simulink model "sg_PID_float"  (Simulink 7.8)
settings: Solver=FixedStepDiscrete  SolverMode=SingleTasking  StartTime=0.0  StopTime=1024*II  RelTol=1e-3
PreLoadFcn:
  | sg_PID_float_PreLoadFcn
StopFcn:
  | sg_PID_float_StopFcn
values from neighbouring files (symbols this model uses):
  C = -0.7931    [sg_ClosedLoop_PID_float_PreLoadFcn.m]    (also in sg_PID_float_PreLoadFcn.m)
  Gd = 6.0324    [sg_ClosedLoop_PID_float_PreLoadFcn.m]    (also in sg_PID_float_PreLoadFcn.m)
  Gi = 0.5112    [sg_ClosedLoop_PID_float_PreLoadFcn.m]    (also in sg_PID_float_PreLoadFcn.m)
  Gp = 35.3675    [sg_ClosedLoop_PID_float_PreLoadFcn.m]    (also in sg_PID_float_PreLoadFcn.m)
  II = 37+1    (= 38)    [sg_ClosedLoop_PID_float_PreLoadFcn.m]    (also in sg_PID_float_PreLoadFcn.m)
  max_clip = MAX_VAL-1    (= 255)    [sg_ClosedLoop_PID_float_PreLoadFcn.m]    (also in sg_PID_float_PreLoadFcn.m = 63)
  min_clip = -MAX_VAL    (= -256)    [sg_ClosedLoop_PID_float_PreLoadFcn.m]    (also in sg_PID_float_PreLoadFcn.m = -64)
libraries: xbsIndex_r4 x97, dspsrcs4 x1
settings Model: Creator=danieleb  LastModifiedBy=danieleb

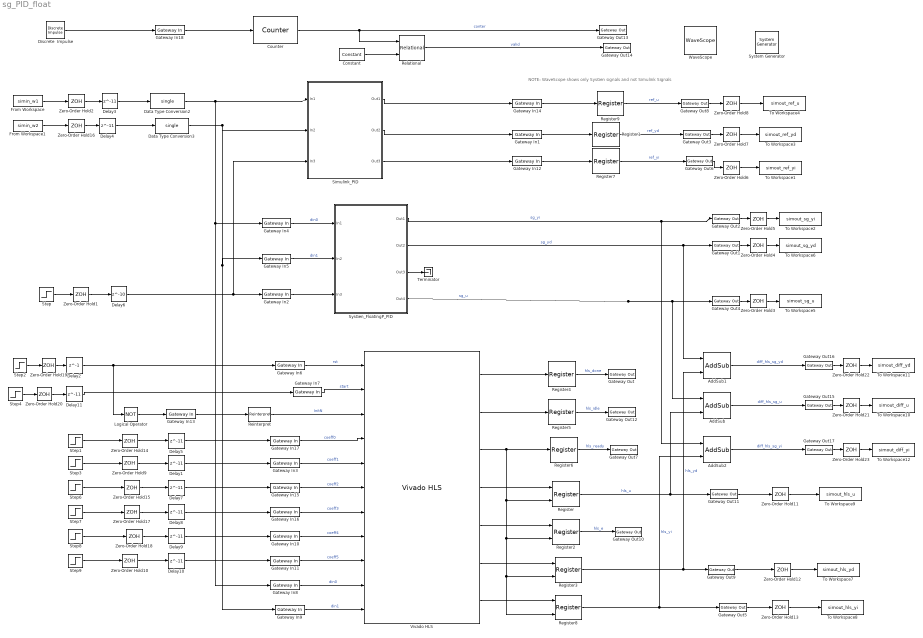
== system sg_PID_float ==
  note: NOTE: WaveScope shows only SysGen signals and not Simulink Signals
  " System Generator" : xbsIndex_r4/ System Generator  Tag=genX  xilinxfamily=zynq  part=xc7z020  speed=-1  package=clg400  synthesis_tool=XST  clock_wrapper=Clock Enables  directory=./netlist_top_PID  proj_type=Project Navigator  Synth_file=XST Defaults  Impl_file=ISE Defaults  testbench=off  simulink_period=1  sysclk_period=10  dcm_input_clock_period=10  incr_netlist=off  trim_vbits=Everywhere in SubSystem  dbl_ovrd=According to Block Masks  core_generation=According to Block Masks  run_coregen=off  deprecated_control=off  eval_field=0  block_type=sysgen
  AddSub : xbsIndex_r4/AddSub  mode=Subtraction  use_carryin=off  use_carryout=off  en=off  latency=0  precision=Full  arith_type=Unsigned  n_bits=16  bin_pt=14  quantization=Truncate  overflow=Wrap  dbl_ovrd=off  use_behavioral_HDL=off  hw_selection=Fabric  pipelined=off  block_type=addsub
  AddSub1 : xbsIndex_r4/AddSub  mode=Subtraction  use_carryin=off  use_carryout=off  en=off  latency=0  precision=Full  arith_type=Unsigned  n_bits=16  bin_pt=14  quantization=Truncate  overflow=Wrap  dbl_ovrd=off  use_behavioral_HDL=off  hw_selection=Fabric  pipelined=off  block_type=addsub
  AddSub2 : xbsIndex_r4/AddSub  mode=Subtraction  use_carryin=off  use_carryout=off  en=off  latency=0  precision=Full  arith_type=Unsigned  n_bits=16  bin_pt=14  quantization=Truncate  overflow=Wrap  dbl_ovrd=off  use_behavioral_HDL=off  hw_selection=Fabric  pipelined=off  block_type=addsub
  Constant : xbsIndex_r4/Constant  const=II-1  gui_display_data_type=Fixed-point  arith_type=Unsigned  n_bits=10  bin_pt=0  preci_type=Single  exp_width=8  frac_width=24  explicit_period=on  period=1  equ=P=C  opselect=C  inp2=PCIN>>17  opr=+  inp1=P  carry=CIN  dbl_ovrd=off  block_type=constant
  Counter : xbsIndex_r4/Counter  cnt_type=Count Limited  cnt_to=II-1  operation=Up  start_count=0  cnt_by_val=1  arith_type=Unsigned  n_bits=10  bin_pt=0  load_pin=off  rst=on  en=off  explicit_period=on  period=1  dbl_ovrd=off  use_behavioral_HDL=off  implementation=Fabric  block_type=counter
  Data Type Conversion2 : DataTypeConversion  OutDataTypeStr=single
  Data Type Conversion3 : DataTypeConversion  OutDataTypeStr=single
  Delay{1,3..5,7..11} (9 alike) : Delay  DelayLength=11
  Delay2 : Delay  DelayLength=1
  Delay6 : Delay  DelayLength=10
  Discrete  Impulse : dspsrcs4/Discrete  Impulse  Delay=0  SampleTime=1  FrameSample=1  dataType=double  isSigned=on  wordLen=16  udDataType=sfix(16)  fracBitsMode=Best precision  numFracBits=15  OutDataTypeStr=double  LastOutDataTypeStr=double
  From Workspace : FromWorkspace  VariableName=simin_w1  SampleTime=II  Interpolate=off  OutputAfterFinalValue=Holding final value
  From Workspace1 : FromWorkspace  VariableName=simin_w2  SampleTime=II  Interpolate=off  OutputAfterFinalValue=Holding final value
  Gateway In{1,3..5,8..12,14..17} (13 alike) : xbsIndex_r4/Gateway In  gui_display_data_type=Floating-point  arith_type=Floating-point  n_bits=25  bin_pt=25-10  preci_type=Single  exp_width=8  frac_width=24  quantization="Round  (unbiased: +/- Inf)"  overflow=Saturate  period=II  dbl_ovrd=off  timing_constraint=None  locs_specified=off  LOCs={}  UseAsADC=off  ADCChannel='1'  inherit_from_input=off  hdl_port=on  block_type=gatewayin
  Gateway In{2,6..7,13} (4 alike) : xbsIndex_r4/Gateway In  gui_display_data_type=Boolean  arith_type=Boolean  n_bits=25  bin_pt=25-10  preci_type=Single  exp_width=8  frac_width=24  quantization="Round  (unbiased: +/- Inf)"  overflow=Saturate  period=II  dbl_ovrd=off  timing_constraint=None  locs_specified=off  LOCs={}  UseAsADC=off  ADCChannel='1'  inherit_from_input=off  hdl_port=on  block_type=gatewayin
  Gateway In18 : xbsIndex_r4/Gateway In  gui_display_data_type=Boolean  arith_type=Boolean  n_bits=25  bin_pt=25-10  preci_type=Single  exp_width=8  frac_width=24  quantization="Round  (unbiased: +/- Inf)"  overflow=Saturate  period=1  dbl_ovrd=off  timing_constraint=None  locs_specified=off  LOCs={}  UseAsADC=off  ADCChannel='1'  inherit_from_input=off  hdl_port=on  block_type=gatewayin
  Gateway Out{,1..6,8..10,12..17} (16 alike) : xbsIndex_r4/Gateway Out  inherit_from_input=off  hdl_port=off  timing_constraint=None  locs_specified=off  LOCs={}  UseAsDAC=off  DACChannel='1'  block_type=gatewayout
  Gateway Out11 : xbsIndex_r4/Gateway Out  inherit_from_input=off  hdl_port=on  timing_constraint=None  locs_specified=off  LOCs={}  UseAsDAC=off  DACChannel='1'  block_type=gatewayout
  Gateway Out7 : xbsIndex_r4/Gateway Out  inherit_from_input=off  hdl_port=on  timing_constraint=None  locs_specified=off  LOCs={}  UseAsDAC=off  DACChannel='1'  block_type=gatewayout
  Logical Operator : Logic  Operator=NOT  AllPortsSameDT=off  OutDataTypeStr=boolean
  Register{,2..3,8} (4 alike) : xbsIndex_r4/Register  init=0  rst=off  en=on  dbl_ovrd=off  block_type=register
  Register{1,4..7,9} (6 alike) : xbsIndex_r4/Register  init=0  rst=off  en=off  dbl_ovrd=off  block_type=register
  Reinterpret : xbsIndex_r4/Reinterpret  force_arith_type=on  arith_type=Unsigned  force_bin_pt=on  bin_pt=0  block_type=reinterpret
  Relational : xbsIndex_r4/Relational  mode=a=b  en=off  latency=0  dbl_ovrd=off  block_type=relational
  Simulink_PID : Subsystem
  Step : Step  Before=1  After=0  SampleTime=II
  Step1 : Step  After=Gi  SampleTime=II
  Step2 : Step  Before=1  After=0  SampleTime=II
  Step3 : Step  After=Gd  SampleTime=II
  Step4 : Step  SampleTime=II
  Step6 : Step  After=C  SampleTime=II
  Step7 : Step  After=Gp  SampleTime=II
  Step8 : Step  After=max_clip  SampleTime=II
  Step9 : Step  After=min_clip  SampleTime=II
  SysGen_FloatingP_PID : Subsystem
      mask Display:
      | fprintf('','COMMENT: begin icon graphics');
      | patch([0 60 60 0 0 ],[0 0 56 56 0 ],[0.77 0.82 0.91 ]);
      | plot([0 60 60 0 0 ],[0 0 56 56 0 ]);
      | patch([12.2 23.76 31.76 39.76 47.76 31.76 20.2 12.2 ],[36.88 36.88 44.88 36.88 44.88 44.88 44.88 36.88 ],[1 1 1 ]);
      | patch([20.2 31.76 23.76 12.2 20.2 ],[28.88 28.88 36.88 36.88 28.88 ],[0.931 0.946 0.973 ]);
      | patch([12.2 23.76 31.76 20.2 12.2 ],[20.88 20.88 28.88 28.88 20.88 ],[1 1 1 ]);
      | patch([20.2 47.76 39.76 31.76 23.76 12.2 20.2 ],[12.88 12.88 20.88 12.88 20.88 20.88 12.88 ],[0.931 0.946 0.973 ]);
      | fprintf('','COMMENT: end icon graphics');
      | fprintf('','COMMENT: begin icon text');
      | color('black');port_label('input',1,' in1');
      | color('black');port_label('input',2,' in2');
      | color('black');port_label('input',3,' rst');
      | color('black');port_label('output',1,'out_i ');
      | color('black');port_label('output',2,'out_d ');
      | color('black');port_label('output',3,'out_p ');
      | color('black');port_label('output',4,'out_u ');
      | fprintf('','COMMENT: end icon text');
  Terminator : Terminator
  To Workspace1 : ToWorkspace  VariableName=simout_ref_yi  SampleTime=-1  SaveFormat=Array
  To Workspace10 : ToWorkspace  VariableName=simout_diff_u  SampleTime=-1  SaveFormat=Array
  To Workspace11 : ToWorkspace  VariableName=simout_diff_yd  SampleTime=-1  SaveFormat=Array
  To Workspace12 : ToWorkspace  VariableName=simout_diff_yi  SampleTime=-1  SaveFormat=Array
  To Workspace2 : ToWorkspace  VariableName=simout_sg_yi  SampleTime=-1  SaveFormat=Array
  To Workspace3 : ToWorkspace  VariableName=simout_ref_yd  SampleTime=-1  SaveFormat=Array
  To Workspace4 : ToWorkspace  VariableName=simout_ref_u  SampleTime=-1  SaveFormat=Array
  To Workspace5 : ToWorkspace  VariableName=simout_sg_u  SampleTime=-1  SaveFormat=Array
  To Workspace6 : ToWorkspace  VariableName=simout_sg_yd  SampleTime=-1  SaveFormat=Array
  To Workspace7 : ToWorkspace  VariableName=simout_hls_yd  SampleTime=-1  SaveFormat=Array
  To Workspace8 : ToWorkspace  VariableName=simout_hls_yi  SampleTime=-1  SaveFormat=Array
  To Workspace9 : ToWorkspace  VariableName=simout_hls_u  SampleTime=-1  SaveFormat=Array
  Vivado HLS : xbsIndex_r4/Vivado HLS  anytable='C:/BagniD/work/xapp_pid/hls/floatp/hls_floatp_pid_prj/solution3_test/'  display_datatype=off  rate_propagation_method=Simulink system period  model_file_path=''  latency=1  block_type=hls
      settings: infoedit=This block allows including C,C++ and SystemC source files in System Generator for DSP designs.
  WaveScope : xbsIndex_r4/WaveScope  block_type=wavescope
  Zero-Order Hold{1..8,11..13,16,19..23} (17 alike) : ZeroOrderHold  SampleTime=II
  Zero-Order Hold{9..10,14..15,17..18} (6 alike) : ZeroOrderHold  SampleTime=-1
  wires:
  Gateway In4/1 -> SysGen_FloatingP_PID/1(In1)  "din0"
  Gateway In5/1 -> SysGen_FloatingP_PID/2(In2)  "din1"
  Register7/1 -> Gateway Out6/1  "ref_yi"
  Gateway In12/1 -> Register7/1
  Gateway Out6/1 -> Zero-Order Hold6/1
  Gateway Out8/1 -> Zero-Order Hold8/1
  Gateway In14/1 -> Register9/1
  Simulink_PID/1(Out1) -> Gateway In14/1
  Register9/1 -> Gateway Out8/1  "ref_u"
  Gateway Out1/1 -> Zero-Order Hold4/1
  Gateway Out2/1 -> Zero-Order Hold5/1
  Gateway Out4/1 -> Zero-Order Hold3/1
  SysGen_FloatingP_PID/4(Out4) -> Gateway Out4/1, AddSub/1  "sg_u"
  Data Type Conversion2/1 -> Gateway In4/1, Gateway In8/1, Simulink_PID/1(In1)
  Data Type Conversion3/1 -> Gateway In5/1, Gateway In9/1, Simulink_PID/2(In2)
  SysGen_FloatingP_PID/1(Out1) -> Gateway Out2/1, AddSub2/1  "sg_yi"
  SysGen_FloatingP_PID/2(Out2) -> Gateway Out1/1, AddSub1/1  "sg_yd"
  SysGen_FloatingP_PID/3(Out3) -> Terminator/1
  Register1/1 -> Gateway Out3/1  "ref_yd"
  Gateway Out3/1 -> Zero-Order Hold7/1
  Gateway In1/1 -> Register1/1
  Gateway In2/1 -> SysGen_FloatingP_PID/3(In3)
  Step/1 -> Zero-Order Hold1/1
  Zero-Order Hold1/1 -> Delay6/1
  Delay6/1 -> Gateway In2/1, Simulink_PID/3(In3)
  Delay3/1 -> Data Type Conversion2/1
  Zero-Order Hold16/1 -> Delay4/1
  Delay4/1 -> Data Type Conversion3/1
  Zero-Order Hold2/1 -> Delay3/1
  From Workspace/1 -> Zero-Order Hold2/1
  From Workspace1/1 -> Zero-Order Hold16/1
  Zero-Order Hold3/1 -> To Workspace5/1
  Zero-Order Hold4/1 -> To Workspace6/1
  Zero-Order Hold5/1 -> To Workspace2/1
  Zero-Order Hold6/1 -> To Workspace1/1
  Zero-Order Hold7/1 -> To Workspace3/1
  Zero-Order Hold8/1 -> To Workspace4/1
  Gateway In6/1 -> Vivado HLS/1  "rst"
  Delay2/1 -> Gateway In6/1, Logical Operator/1
  Delay11/1 -> Gateway In7/1
  Delay5/1 -> Gateway In17/1
  Gateway In17/1 -> Vivado HLS/4  "coeff0"
  Gateway In7/1 -> Vivado HLS/2  "start"
  Reinterpret/1 -> Vivado HLS/3  "InitN"
  Zero-Order Hold14/1 -> Delay5/1
  Step1/1 -> Zero-Order Hold14/1
  Delay1/1 -> Gateway In3/1
  Gateway In3/1 -> Vivado HLS/5  "coeff1"
  Zero-Order Hold9/1 -> Delay1/1
  Step3/1 -> Zero-Order Hold9/1
  Gateway In8/1 -> Vivado HLS/10  "din0"
  Gateway In9/1 -> Vivado HLS/11  "din1"
  Gateway In13/1 -> Reinterpret/1
  Logical Operator/1 -> Gateway In13/1
  Gateway In15/1 -> Vivado HLS/6  "coeff2"
  Gateway In16/1 -> Vivado HLS/7  "coeff3"
  Gateway In10/1 -> Vivado HLS/8  "coeff4"
  Gateway In11/1 -> Vivado HLS/9  "coeff5"
  Delay7/1 -> Gateway In15/1
  Delay8/1 -> Gateway In16/1
  Delay9/1 -> Gateway In10/1
  Delay10/1 -> Gateway In11/1
  Zero-Order Hold15/1 -> Delay7/1
  Zero-Order Hold17/1 -> Delay8/1
  Step6/1 -> Zero-Order Hold15/1
  Step7/1 -> Zero-Order Hold17/1
  Zero-Order Hold18/1 -> Delay9/1
  Step8/1 -> Zero-Order Hold18/1
  Zero-Order Hold10/1 -> Delay10/1
  Step9/1 -> Zero-Order Hold10/1
  Register/1 -> Gateway Out11/1, AddSub/2  "hls_u"
  Register2/1 -> Gateway Out10/1  "hls_e"
  Register3/1 -> Gateway Out9/1, AddSub1/2  "hls_yd"
  Register4/1 -> Gateway Out/1  "hls_done"
  Register5/1 -> Gateway Out12/1  "hls_idle"
  Register6/1 -> Gateway Out7/1  "hls_ready"
  Register8/1 -> Gateway Out5/1, AddSub2/2  "hls_yi"
  Gateway Out9/1 -> Zero-Order Hold12/1
  Gateway Out5/1 -> Zero-Order Hold13/1
  Gateway Out11/1 -> Zero-Order Hold11/1
  Vivado HLS/1 -> Register4/1
  Vivado HLS/2 -> Register5/1
  Vivado HLS/3 -> Register6/1, Register/2, Register2/2, Register3/2, Register8/2
  Vivado HLS/4 -> Register/1
  Vivado HLS/5 -> Register2/1
  Vivado HLS/6 -> Register3/1
  Vivado HLS/7 -> Register8/1
  Zero-Order Hold11/1 -> To Workspace9/1
  Zero-Order Hold12/1 -> To Workspace7/1
  Zero-Order Hold13/1 -> To Workspace8/1
  Step2/1 -> Zero-Order Hold19/1
  Zero-Order Hold19/1 -> Delay2/1
  Step4/1 -> Zero-Order Hold20/1
  Zero-Order Hold20/1 -> Delay11/1
  Gateway In18/1 -> Counter/1
  Discrete  Impulse/1 -> Gateway In18/1
  Counter/1 -> Gateway Out13/1, Relational/1  "conter"
  Constant/1 -> Relational/2
  Relational/1 -> Gateway Out14/1  "valid"
  Gateway Out15/1 -> Zero-Order Hold21/1
  AddSub/1 -> Gateway Out15/1  "diff_hls_sg_u"
  Zero-Order Hold21/1 -> To Workspace10/1
  Gateway Out16/1 -> Zero-Order Hold22/1
  AddSub1/1 -> Gateway Out16/1  "diff_hls_sg_yd"
  Zero-Order Hold22/1 -> To Workspace11/1
  Gateway Out17/1 -> Zero-Order Hold23/1
  AddSub2/1 -> Gateway Out17/1  "diff_hls_sg_yi"
  Zero-Order Hold23/1 -> To Workspace12/1
  Simulink_PID/2(Out2) -> Gateway In1/1
  Simulink_PID/3(Out3) -> Gateway In12/1

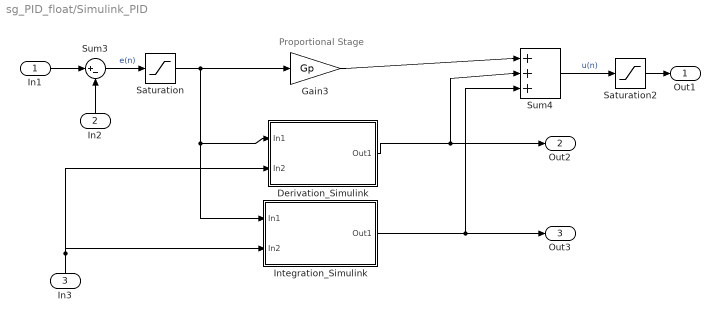
== system sg_PID_float/Simulink_PID ==
  note: Proportional Stage
  In1 : Inport
  In2 : Inport  Port=2
  In3 : Inport  Port=3
  Derivation_Simulink : Subsystem
  Gain3 : Gain  Gain=Gp
  Integration_Simulink : Subsystem
  Saturation : Saturate  UpperLimit=max_clip  LowerLimit=min_clip
  Saturation2 : Saturate  UpperLimit=max_clip  LowerLimit=min_clip
  Sum3 : Sum  Inputs=|+-
  Sum4 : Sum  Inputs=|+++
  Out1 : Outport
  Out2 : Outport  Port=2
  Out3 : Outport  Port=3
  wires:
  Gain3/1 -> Sum4/1
  Sum3/1 -> Saturation/1  "e(n)"
  Sum4/1 -> Saturation2/1  "u(n)"
  Saturation/1 -> Gain3/1, Derivation_Simulink/1(In1), Integration_Simulink/1(In1)
  Derivation_Simulink/1(Out1) -> Sum4/2, Out2/1
  Integration_Simulink/1(Out1) -> Sum4/3, Out3/1
  In1/1 -> Sum3/1
  In2/1 -> Sum3/2
  In3/1 -> Integration_Simulink/2(In2), Derivation_Simulink/2(In2)
  Saturation2/1 -> Out1/1

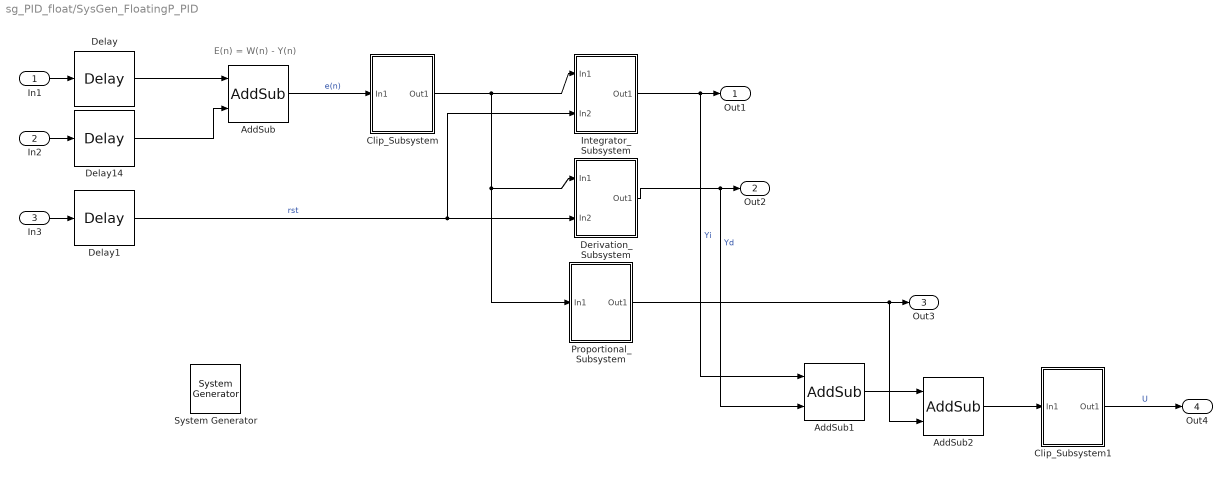
== system sg_PID_float/SysGen_FloatingP_PID ==
  note: E(n) = W(n) - Y(n)
  In1 : Inport
  In2 : Inport  Port=2
  In3 : Inport  Port=3
  " System Generator" : xbsIndex_r4/ System Generator  Tag=genX  xilinxfamily=virtex6  part=xc6vlx240t  speed=-2  package=ff1156  synthesis_tool=XST  clock_wrapper=Clock Enables  directory=./timing_v6lx240t  proj_type=Project Navigator  Synth_file=XST Defaults  Impl_file=ISE Defaults  testbench=off  simulink_period=1  sysclk_period=1.000000e+001  dcm_input_clock_period=10  incr_netlist=off  trim_vbits=Everywhere in SubSystem  dbl_ovrd=According to Block Masks  core_generation=According to Block Masks  run_coregen=off  deprecated_control=off  eval_field=0  block_type=sysgen
  AddSub : xbsIndex_r4/AddSub  mode=Subtraction  use_carryin=off  use_carryout=off  en=off  latency=0  precision=Full  arith_type=Unsigned  n_bits=16  bin_pt=14  quantization=Truncate  overflow=Wrap  dbl_ovrd=off  use_behavioral_HDL=off  hw_selection=DSP48  pipelined=off  block_type=addsub
  AddSub1 : xbsIndex_r4/AddSub  mode=Addition  use_carryin=off  use_carryout=off  en=off  latency=0  precision=Full  arith_type=Unsigned  n_bits=16  bin_pt=14  quantization=Truncate  overflow=Wrap  dbl_ovrd=off  use_behavioral_HDL=off  hw_selection=DSP48  pipelined=off  block_type=addsub
  AddSub2 : xbsIndex_r4/AddSub  mode=Addition  use_carryin=off  use_carryout=off  en=off  latency=0  precision=Full  arith_type=Unsigned  n_bits=16  bin_pt=14  quantization=Truncate  overflow=Wrap  dbl_ovrd=off  use_behavioral_HDL=off  hw_selection=DSP48  pipelined=off  block_type=addsub
  Clip_Subsystem : Subsystem
      mask Display:
      | fprintf('','COMMENT: begin icon graphics');
      | patch([0 60 60 0 0 ],[0 0 58 58 0 ],[0.77 0.82 0.91 ]);
      | plot([0 60 60 0 0 ],[0 0 58 58 0 ]);
      | patch([12.2 23.76 31.76 39.76 47.76 31.76 20.2 12.2 ],[37.88 37.88 45.88 37.88 45.88 45.88 45.88 37.88 ],[1 1 1 ]);
      | patch([20.2 31.76 23.76 12.2 20.2 ],[29.88 29.88 37.88 37.88 29.88 ],[0.931 0.946 0.973 ]);
      | patch([12.2 23.76 31.76 20.2 12.2 ],[21.88 21.88 29.88 29.88 21.88 ],[1 1 1 ]);
      | patch([20.2 47.76 39.76 31.76 23.76 12.2 20.2 ],[13.88 13.88 21.88 13.88 21.88 21.88 13.88 ],[0.931 0.946 0.973 ]);
      | fprintf('','COMMENT: end icon graphics');
      | fprintf('','COMMENT: begin icon text');
      | color('black');port_label('input',1,' Din');
      | color('black');port_label('output',1,'Dout ');
      | fprintf('','COMMENT: end icon text');
  Clip_Subsystem1 : Subsystem
      mask Display:
      | fprintf('','COMMENT: begin icon graphics');
      | patch([0 60 60 0 0 ],[0 0 58 58 0 ],[0.77 0.82 0.91 ]);
      | plot([0 60 60 0 0 ],[0 0 58 58 0 ]);
      | patch([12.2 23.76 31.76 39.76 47.76 31.76 20.2 12.2 ],[37.88 37.88 45.88 37.88 45.88 45.88 45.88 37.88 ],[1 1 1 ]);
      | patch([20.2 31.76 23.76 12.2 20.2 ],[29.88 29.88 37.88 37.88 29.88 ],[0.931 0.946 0.973 ]);
      | patch([12.2 23.76 31.76 20.2 12.2 ],[21.88 21.88 29.88 29.88 21.88 ],[1 1 1 ]);
      | patch([20.2 47.76 39.76 31.76 23.76 12.2 20.2 ],[13.88 13.88 21.88 13.88 21.88 21.88 13.88 ],[0.931 0.946 0.973 ]);
      | fprintf('','COMMENT: end icon graphics');
      | fprintf('','COMMENT: begin icon text');
      | color('black');port_label('input',1,' Din');
      | color('black');port_label('output',1,'Dout ');
      | fprintf('','COMMENT: end icon text');
  Delay : xbsIndex_r4/Delay  rst=off  infoeditControl=Selection of Reset will increase slice count due to use of real FFs and instead of SRLs  en=off  latency=1  dbl_ovrd=off  reg_retiming=off  block_type=delay
  Delay1 : xbsIndex_r4/Delay  rst=off  infoeditControl=Selection of Reset will increase slice count due to use of real FFs and instead of SRLs  en=off  latency=1  dbl_ovrd=off  reg_retiming=off  block_type=delay
  Delay14 : xbsIndex_r4/Delay  rst=off  infoeditControl=Selection of Reset will increase slice count due to use of real FFs and instead of SRLs  en=off  latency=1  dbl_ovrd=off  reg_retiming=off  block_type=delay
  Derivation_Subsystem : Subsystem
      mask Display:
      | fprintf('','COMMENT: begin icon graphics');
      | patch([0 60 60 0 0 ],[0 0 58 58 0 ],[0.77 0.82 0.91 ]);
      | plot([0 60 60 0 0 ],[0 0 58 58 0 ]);
      | patch([12.2 23.76 31.76 39.76 47.76 31.76 20.2 12.2 ],[37.88 37.88 45.88 37.88 45.88 45.88 45.88 37.88 ],[1 1 1 ]);
      | patch([20.2 31.76 23.76 12.2 20.2 ],[29.88 29.88 37.88 37.88 29.88 ],[0.931 0.946 0.973 ]);
      | patch([12.2 23.76 31.76 20.2 12.2 ],[21.88 21.88 29.88 29.88 21.88 ],[1 1 1 ]);
      | patch([20.2 47.76 39.76 31.76 23.76 12.2 20.2 ],[13.88 13.88 21.88 13.88 21.88 21.88 13.88 ],[0.931 0.946 0.973 ]);
      | fprintf('','COMMENT: end icon graphics');
      | fprintf('','COMMENT: begin icon text');
      | color('black');port_label('input',1,' X1');
      | color('black');port_label('output',1,'Yd ');
      | fprintf('','COMMENT: end icon text');
  Integrator_Subsystem : Subsystem
      mask Display:
      | fprintf('','COMMENT: begin icon graphics');
      | patch([0 60 60 0 0 ],[0 0 58 58 0 ],[0.77 0.82 0.91 ]);
      | plot([0 60 60 0 0 ],[0 0 58 58 0 ]);
      | patch([12.2 23.76 31.76 39.76 47.76 31.76 20.2 12.2 ],[37.88 37.88 45.88 37.88 45.88 45.88 45.88 37.88 ],[1 1 1 ]);
      | patch([20.2 31.76 23.76 12.2 20.2 ],[29.88 29.88 37.88 37.88 29.88 ],[0.931 0.946 0.973 ]);
      | patch([12.2 23.76 31.76 20.2 12.2 ],[21.88 21.88 29.88 29.88 21.88 ],[1 1 1 ]);
      | patch([20.2 47.76 39.76 31.76 23.76 12.2 20.2 ],[13.88 13.88 21.88 13.88 21.88 21.88 13.88 ],[0.931 0.946 0.973 ]);
      | fprintf('','COMMENT: end icon graphics');
      | fprintf('','COMMENT: begin icon text');
      | color('black');port_label('input',1,' X2');
      | color('black');port_label('output',1,'Yi ');
      | fprintf('','COMMENT: end icon text');
  Proportional_Subsystem : Subsystem
      mask Display:
      | fprintf('','COMMENT: begin icon graphics');
      | patch([0 60 60 0 0 ],[0 0 58 58 0 ],[0.77 0.82 0.91 ]);
      | plot([0 60 60 0 0 ],[0 0 58 58 0 ]);
      | patch([12.2 23.76 31.76 39.76 47.76 31.76 20.2 12.2 ],[37.88 37.88 45.88 37.88 45.88 45.88 45.88 37.88 ],[1 1 1 ]);
      | patch([20.2 31.76 23.76 12.2 20.2 ],[29.88 29.88 37.88 37.88 29.88 ],[0.931 0.946 0.973 ]);
      | patch([12.2 23.76 31.76 20.2 12.2 ],[21.88 21.88 29.88 29.88 21.88 ],[1 1 1 ]);
      | patch([20.2 47.76 39.76 31.76 23.76 12.2 20.2 ],[13.88 13.88 21.88 13.88 21.88 21.88 13.88 ],[0.931 0.946 0.973 ]);
      | fprintf('','COMMENT: end icon graphics');
      | fprintf('','COMMENT: begin icon text');
      | color('black');port_label('input',1,' X');
      | color('black');port_label('output',1,'Y ');
      | fprintf('','COMMENT: end icon text');
  Out1 : Outport
  Out2 : Outport  Port=2
  Out3 : Outport  Port=3
  Out4 : Outport  Port=4
  wires:
  Delay/1 -> AddSub/1
  Delay14/1 -> AddSub/2
  AddSub/1 -> Clip_Subsystem/1(In1)  "e(n)"
  Clip_Subsystem/1(Out1) -> Integrator_Subsystem/1(In1), Derivation_Subsystem/1(In1), Proportional_Subsystem/1(In1)
  Derivation_Subsystem/1(Out1) -> AddSub1/2, Out2/1  "Yd"
  Integrator_Subsystem/1(Out1) -> AddSub1/1, Out1/1  "Yi"
  Proportional_Subsystem/1(Out1) -> AddSub2/2, Out3/1
  AddSub1/1 -> AddSub2/1
  AddSub2/1 -> Clip_Subsystem1/1(In1)
  In1/1 -> Delay/1
  In2/1 -> Delay14/1
  Clip_Subsystem1/1(Out1) -> Out4/1  "U"
  In3/1 -> Delay1/1
  Delay1/1 -> Integrator_Subsystem/2(In2), Derivation_Subsystem/2(In2)  "rst"

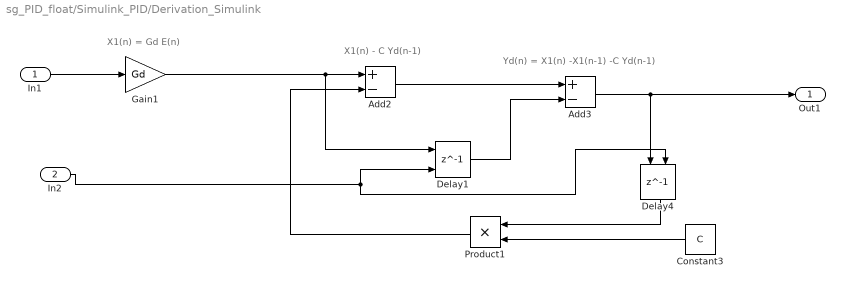
== system sg_PID_float/Simulink_PID/Derivation_Simulink ==
  note: X1(n) - C Yd(n-1)
  note: Yd(n) = X1(n) -X1(n-1) -C Yd(n-1)
  note: X1(n) = Gd E(n)
  In1 : Inport
  In2 : Inport  Port=2
  Add2 : Sum  Inputs=+-
  Add3 : Sum  Inputs=+-
  Constant3 : Constant  Value=C  OutDataTypeStr=single  SampleTime=II
  Delay1 : Delay  DelayLength=1  ExternalReset=Level hold
      settings: InputPortMap=u0,r5
  Delay4 : Delay  DelayLength=1  ExternalReset=Level hold
      settings: InputPortMap=u0,r5
  Gain1 : Gain  Gain=Gd
  Product1 : Product  RndMeth=Zero
  Out1 : Outport
  wires:
  In1/1 -> Gain1/1
  Delay1/1 -> Add3/2
  Add2/1 -> Add3/1
  Add3/1 -> Delay4/1, Out1/1
  Constant3/1 -> Product1/2
  Product1/1 -> Add2/2
  Delay4/1 -> Product1/1
  In2/1 -> Delay1/2, Delay4/2
  Gain1/1 -> Add2/1, Delay1/1

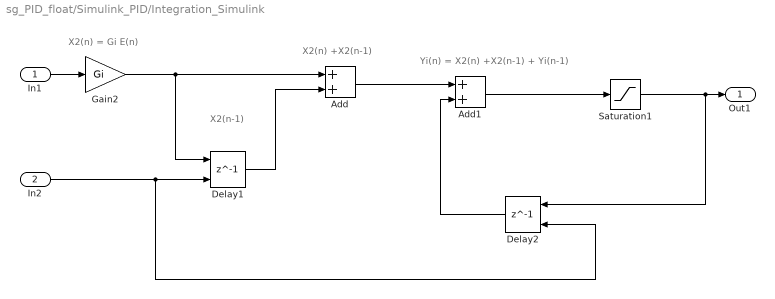
== system sg_PID_float/Simulink_PID/Integration_Simulink ==
  note: X2(n) = Gi E(n)
  note: X2(n) +X2(n-1)
  note: X2(n-1)
  note: Yi(n) = X2(n) +X2(n-1) + Yi(n-1)
  In1 : Inport
  In2 : Inport  Port=2
  Add : Sum
  Add1 : Sum
  Delay1 : Delay  DelayLength=1  ExternalReset=Level hold
      settings: InputPortMap=u0,r5
  Delay2 : Delay  DelayLength=1  ExternalReset=Level hold
      settings: InputPortMap=u0,r5
  Gain2 : Gain  Gain=Gi
  Saturation1 : Saturate  UpperLimit=max_clip  LowerLimit=min_clip
  Out1 : Outport
  wires:
  Add/1 -> Add1/1
  Add1/1 -> Saturation1/1
  Gain2/1 -> Add/1, Delay1/1
  Delay1/1 -> Add/2
  Saturation1/1 -> Out1/1, Delay2/1
  In1/1 -> Gain2/1
  Delay2/1 -> Add1/2
  In2/1 -> Delay1/2, Delay2/2

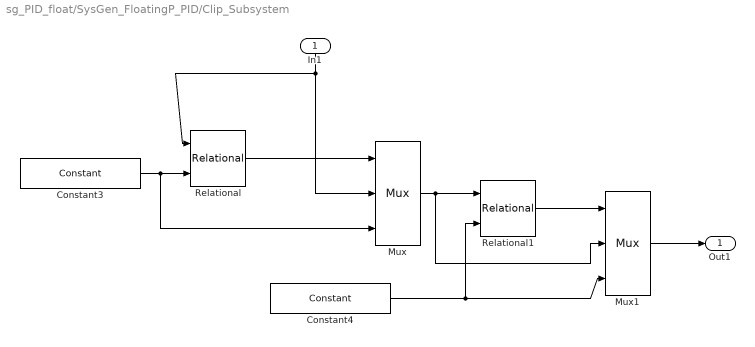
== system sg_PID_float/SysGen_FloatingP_PID/Clip_Subsystem ==
  In1 : Inport
  Constant3 : xbsIndex_r4/Constant  const=max_clip  gui_display_data_type=Floating-point  arith_type=Floating-point  n_bits=16  bin_pt=14  preci_type=Single  exp_width=8  frac_width=24  explicit_period=on  period=II  equ=P=C  opselect=C  inp2=PCIN>>17  opr=+  inp1=P  carry=CIN  dbl_ovrd=off  block_type=constant
  Constant4 : xbsIndex_r4/Constant  const=min_clip  gui_display_data_type=Floating-point  arith_type=Floating-point  n_bits=16  bin_pt=14  preci_type=Single  exp_width=8  frac_width=24  explicit_period=on  period=II  equ=P=C  opselect=C  inp2=PCIN>>17  opr=+  inp1=P  carry=CIN  dbl_ovrd=off  block_type=constant
  Mux : xbsIndex_r4/Mux  inputs=2  en=off  latency=0  precision=Full  arith_type=Unsigned  n_bits=16  bin_pt=14  quantization=Truncate  overflow=Wrap  dbl_ovrd=off  block_type=mux
  Mux1 : xbsIndex_r4/Mux  inputs=2  en=off  latency=0  precision=Full  arith_type=Unsigned  n_bits=16  bin_pt=14  quantization=Truncate  overflow=Wrap  dbl_ovrd=off  block_type=mux
  Relational : xbsIndex_r4/Relational  mode=a>=b  en=off  latency=0  dbl_ovrd=off  block_type=relational
  Relational1 : xbsIndex_r4/Relational  mode=a<=b  en=off  latency=0  dbl_ovrd=off  block_type=relational
  Out1 : Outport
  wires:
  Constant3/1 -> Relational/2, Mux/3
  Relational/1 -> Mux/1
  In1/1 -> Relational/1, Mux/2
  Mux/1 -> Relational1/1, Mux1/2
  Constant4/1 -> Mux1/3, Relational1/2
  Relational1/1 -> Mux1/1
  Mux1/1 -> Out1/1

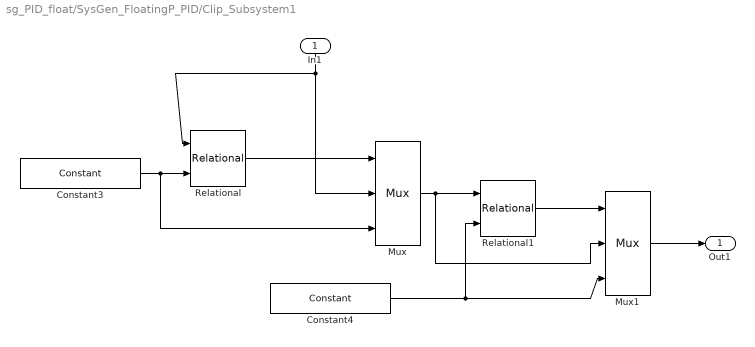
== system sg_PID_float/SysGen_FloatingP_PID/Clip_Subsystem1 ==
  In1 : Inport
  Constant3 : xbsIndex_r4/Constant  const=max_clip  gui_display_data_type=Floating-point  arith_type=Floating-point  n_bits=16  bin_pt=14  preci_type=Single  exp_width=8  frac_width=24  explicit_period=on  period=II  equ=P=C  opselect=C  inp2=PCIN>>17  opr=+  inp1=P  carry=CIN  dbl_ovrd=off  block_type=constant
  Constant4 : xbsIndex_r4/Constant  const=min_clip  gui_display_data_type=Floating-point  arith_type=Floating-point  n_bits=16  bin_pt=14  preci_type=Single  exp_width=8  frac_width=24  explicit_period=on  period=II  equ=P=C  opselect=C  inp2=PCIN>>17  opr=+  inp1=P  carry=CIN  dbl_ovrd=off  block_type=constant
  Mux : xbsIndex_r4/Mux  inputs=2  en=off  latency=0  precision=Full  arith_type=Unsigned  n_bits=16  bin_pt=14  quantization=Truncate  overflow=Wrap  dbl_ovrd=off  block_type=mux
  Mux1 : xbsIndex_r4/Mux  inputs=2  en=off  latency=0  precision=Full  arith_type=Unsigned  n_bits=16  bin_pt=14  quantization=Truncate  overflow=Wrap  dbl_ovrd=off  block_type=mux
  Relational : xbsIndex_r4/Relational  mode=a>=b  en=off  latency=0  dbl_ovrd=off  block_type=relational
  Relational1 : xbsIndex_r4/Relational  mode=a<=b  en=off  latency=0  dbl_ovrd=off  block_type=relational
  Out1 : Outport
  wires:
  Mux1/1 -> Out1/1
  Relational1/1 -> Mux1/1
  Constant4/1 -> Relational1/2, Mux1/3
  Mux/1 -> Mux1/2, Relational1/1
  In1/1 -> Mux/2, Relational/1
  Relational/1 -> Mux/1
  Constant3/1 -> Mux/3, Relational/2

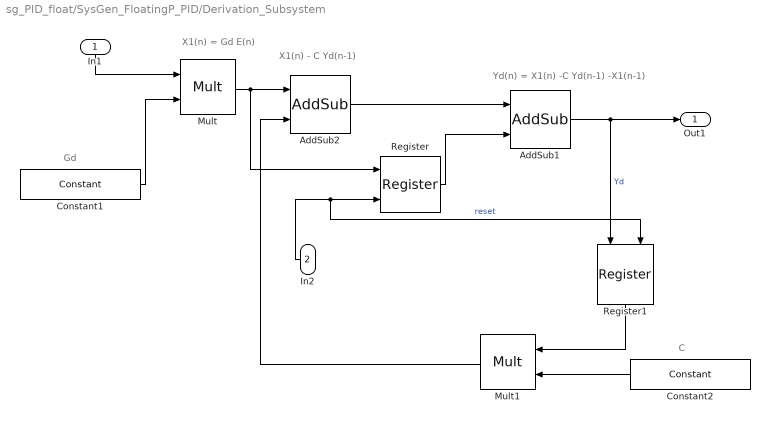
== system sg_PID_float/SysGen_FloatingP_PID/Derivation_Subsystem ==
  note: X1(n) - C Yd(n-1)
  note: Yd(n) = X1(n) -C Yd(n-1) -X1(n-1)
  note: X1(n) = Gd E(n)
  note: Gd
  note: C
  In1 : Inport
  In2 : Inport  Port=2
  AddSub1 : xbsIndex_r4/AddSub  mode=Subtraction  use_carryin=off  use_carryout=off  en=off  latency=0  precision=Full  arith_type=Unsigned  n_bits=16  bin_pt=14  quantization=Truncate  overflow=Wrap  dbl_ovrd=off  use_behavioral_HDL=off  hw_selection=Fabric  pipelined=off  block_type=addsub
  AddSub2 : xbsIndex_r4/AddSub  mode=Subtraction  use_carryin=off  use_carryout=off  en=off  latency=0  precision=Full  arith_type=Unsigned  n_bits=16  bin_pt=14  quantization=Truncate  overflow=Wrap  dbl_ovrd=off  use_behavioral_HDL=off  hw_selection=Fabric  pipelined=off  block_type=addsub
  Constant1 : xbsIndex_r4/Constant  const=Gd  gui_display_data_type=Floating-point  arith_type=Floating-point  n_bits=16  bin_pt=14  preci_type=Single  exp_width=8  frac_width=24  explicit_period=on  period=II  equ=P=C  opselect=C  inp2=PCIN>>17  opr=+  inp1=P  carry=CIN  dbl_ovrd=off  block_type=constant
  Constant2 : xbsIndex_r4/Constant  const=C  gui_display_data_type=Floating-point  arith_type=Floating-point  n_bits=16  bin_pt=14  preci_type=Single  exp_width=8  frac_width=24  explicit_period=on  period=II  equ=P=C  opselect=C  inp2=PCIN>>17  opr=+  inp1=P  carry=CIN  dbl_ovrd=off  block_type=constant
  Mult : xbsIndex_r4/Mult  precision=Full  arith_type="Signed  (2's comp)"  n_bits=16  bin_pt=14  quantization=Truncate  overflow=Wrap  en=off  latency=0  dbl_ovrd=off  use_behavioral_HDL=off  opt=Speed  use_embedded=on  optimum_pipeline=off  pipeline=on  use_rpm=on  placement_style=Triangular  block_type=mult
  Mult1 : xbsIndex_r4/Mult  precision=Full  arith_type="Signed  (2's comp)"  n_bits=16  bin_pt=14  quantization=Truncate  overflow=Wrap  en=off  latency=0  dbl_ovrd=off  use_behavioral_HDL=off  opt=Speed  use_embedded=on  optimum_pipeline=off  pipeline=on  use_rpm=on  placement_style=Triangular  block_type=mult
  Register : xbsIndex_r4/Register  init=0  rst=on  en=off  dbl_ovrd=off  block_type=register
  Register1 : xbsIndex_r4/Register  init=0  rst=on  en=off  dbl_ovrd=off  block_type=register
  Out1 : Outport
  wires:
  In1/1 -> Mult/1
  AddSub2/1 -> AddSub1/1
  Mult/1 -> AddSub2/1, Register/1
  Mult1/1 -> AddSub2/2
  Constant2/1 -> Mult1/2
  AddSub1/1 -> Out1/1, Register1/1  "Yd"
  Register/1 -> AddSub1/2
  Constant1/1 -> Mult/2
  Register1/1 -> Mult1/1
  In2/1 -> Register/2, Register1/2  "reset"

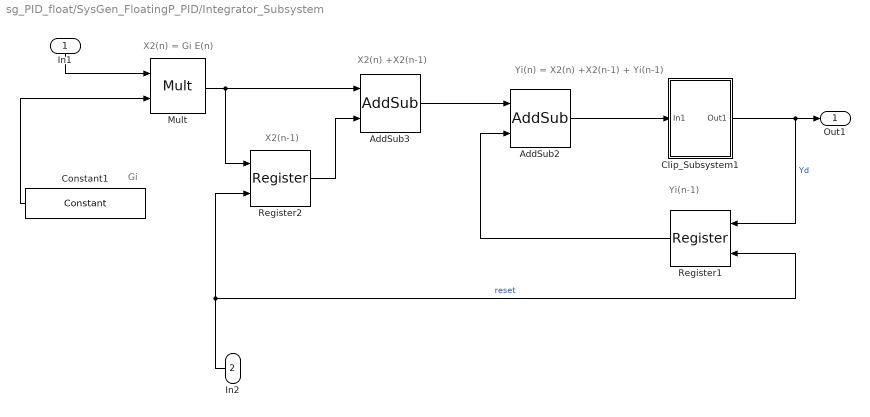
== system sg_PID_float/SysGen_FloatingP_PID/Integrator_Subsystem ==
  note: X2(n) = Gi E(n)
  note: Yi(n) = X2(n) +X2(n-1) + Yi(n-1)
  note: X2(n) +X2(n-1)
  note: X2(n-1)
  note: Yi(n-1)
  note: Gi
  In1 : Inport
  In2 : Inport  Port=2
  AddSub2 : xbsIndex_r4/AddSub  mode=Addition  use_carryin=off  use_carryout=off  en=off  latency=0  precision=Full  arith_type=Unsigned  n_bits=16  bin_pt=14  quantization=Truncate  overflow=Wrap  dbl_ovrd=off  use_behavioral_HDL=off  hw_selection=DSP48  pipelined=off  block_type=addsub
  AddSub3 : xbsIndex_r4/AddSub  mode=Addition  use_carryin=off  use_carryout=off  en=off  latency=0  precision=Full  arith_type=Unsigned  n_bits=16  bin_pt=14  quantization=Truncate  overflow=Wrap  dbl_ovrd=off  use_behavioral_HDL=off  hw_selection=DSP48  pipelined=off  block_type=addsub
  Clip_Subsystem1 : Subsystem
      mask Display:
      | fprintf('','COMMENT: begin icon graphics');
      | patch([0 60 60 0 0 ],[0 0 58 58 0 ],[0.77 0.82 0.91 ]);
      | plot([0 60 60 0 0 ],[0 0 58 58 0 ]);
      | patch([12.2 23.76 31.76 39.76 47.76 31.76 20.2 12.2 ],[37.88 37.88 45.88 37.88 45.88 45.88 45.88 37.88 ],[1 1 1 ]);
      | patch([20.2 31.76 23.76 12.2 20.2 ],[29.88 29.88 37.88 37.88 29.88 ],[0.931 0.946 0.973 ]);
      | patch([12.2 23.76 31.76 20.2 12.2 ],[21.88 21.88 29.88 29.88 21.88 ],[1 1 1 ]);
      | patch([20.2 47.76 39.76 31.76 23.76 12.2 20.2 ],[13.88 13.88 21.88 13.88 21.88 21.88 13.88 ],[0.931 0.946 0.973 ]);
      | fprintf('','COMMENT: end icon graphics');
      | fprintf('','COMMENT: begin icon text');
      | color('black');port_label('input',1,' Din');
      | color('black');port_label('output',1,'Dout ');
      | fprintf('','COMMENT: end icon text');
  Constant1 : xbsIndex_r4/Constant  const=Gi  gui_display_data_type=Floating-point  arith_type=Floating-point  n_bits=16  bin_pt=14  preci_type=Single  exp_width=8  frac_width=24  explicit_period=on  period=II  equ=P=C  opselect=C  inp2=PCIN>>17  opr=+  inp1=P  carry=CIN  dbl_ovrd=off  block_type=constant
  Mult : xbsIndex_r4/Mult  precision=Full  arith_type="Signed  (2's comp)"  n_bits=16  bin_pt=14  quantization=Truncate  overflow=Wrap  en=off  latency=0  dbl_ovrd=off  use_behavioral_HDL=off  opt=Speed  use_embedded=on  optimum_pipeline=off  pipeline=on  use_rpm=on  placement_style=Triangular  block_type=mult
  Register1 : xbsIndex_r4/Register  init=0  rst=on  en=off  dbl_ovrd=off  block_type=register
  Register2 : xbsIndex_r4/Register  init=0  rst=on  en=off  dbl_ovrd=off  block_type=register
  Out1 : Outport
  wires:
  Constant1/1 -> Mult/2
  Clip_Subsystem1/1(Out1) -> Out1/1, Register1/1  "Yd"
  In1/1 -> Mult/1
  Mult/1 -> AddSub3/1, Register2/1
  Register2/1 -> AddSub3/2
  Register1/1 -> AddSub2/2
  AddSub3/1 -> AddSub2/1
  AddSub2/1 -> Clip_Subsystem1/1(In1)
  In2/1 -> Register2/2, Register1/2  "reset"

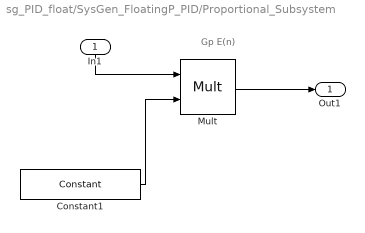
== system sg_PID_float/SysGen_FloatingP_PID/Proportional_Subsystem ==
  note: Gp E(n)
  In1 : Inport
  Constant1 : xbsIndex_r4/Constant  const=Gp  gui_display_data_type=Floating-point  arith_type=Floating-point  n_bits=16  bin_pt=14  preci_type=Single  exp_width=8  frac_width=24  explicit_period=on  period=II  equ=P=C  opselect=C  inp2=PCIN>>17  opr=+  inp1=P  carry=CIN  dbl_ovrd=off  block_type=constant
  Mult : xbsIndex_r4/Mult  precision=Full  arith_type="Signed  (2's comp)"  n_bits=16  bin_pt=14  quantization=Truncate  overflow=Wrap  en=off  latency=0  dbl_ovrd=off  use_behavioral_HDL=off  opt=Speed  use_embedded=on  optimum_pipeline=off  pipeline=on  use_rpm=on  placement_style=Triangular  block_type=mult
  Out1 : Outport
  wires:
  Constant1/1 -> Mult/2
  Mult/1 -> Out1/1
  In1/1 -> Mult/1

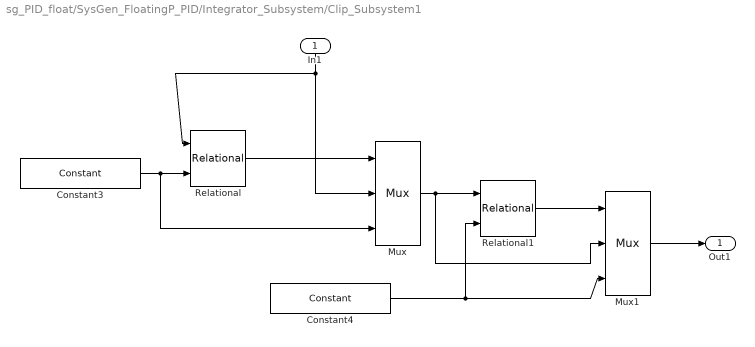
== system sg_PID_float/SysGen_FloatingP_PID/Integrator_Subsystem/Clip_Subsystem1 ==
  In1 : Inport
  Constant3 : xbsIndex_r4/Constant  const=max_clip  gui_display_data_type=Floating-point  arith_type=Floating-point  n_bits=16  bin_pt=14  preci_type=Single  exp_width=8  frac_width=24  explicit_period=on  period=II  equ=P=C  opselect=C  inp2=PCIN>>17  opr=+  inp1=P  carry=CIN  dbl_ovrd=off  block_type=constant
  Constant4 : xbsIndex_r4/Constant  const=min_clip  gui_display_data_type=Floating-point  arith_type=Floating-point  n_bits=16  bin_pt=14  preci_type=Single  exp_width=8  frac_width=24  explicit_period=on  period=II  equ=P=C  opselect=C  inp2=PCIN>>17  opr=+  inp1=P  carry=CIN  dbl_ovrd=off  block_type=constant
  Mux : xbsIndex_r4/Mux  inputs=2  en=off  latency=0  precision=Full  arith_type=Unsigned  n_bits=16  bin_pt=14  quantization=Truncate  overflow=Wrap  dbl_ovrd=off  block_type=mux
  Mux1 : xbsIndex_r4/Mux  inputs=2  en=off  latency=0  precision=Full  arith_type=Unsigned  n_bits=16  bin_pt=14  quantization=Truncate  overflow=Wrap  dbl_ovrd=off  block_type=mux
  Relational : xbsIndex_r4/Relational  mode=a>=b  en=off  latency=0  dbl_ovrd=off  block_type=relational
  Relational1 : xbsIndex_r4/Relational  mode=a<=b  en=off  latency=0  dbl_ovrd=off  block_type=relational
  Out1 : Outport
  wires:
  Mux1/1 -> Out1/1
  Relational1/1 -> Mux1/1
  Constant4/1 -> Relational1/2, Mux1/3
  Mux/1 -> Mux1/2, Relational1/1
  In1/1 -> Mux/2, Relational/1
  Relational/1 -> Mux/1
  Constant3/1 -> Mux/3, Relational/2
